simulink model "Hybridchargingstation"  (R2022a)
settings: Solver=ode23tb  StartTime=0.0  StopTime=20  RelTol=1e-3  EnableMultiTasking=on
undefined symbols (not defined in the file): Ion, Lithium
libraries: spsVoltageMeasurementLib x15, spsSeriesRLCBranchLib x9, spsIdealSwitchLib x9, spsDiodeLib x8, slpidlib x7, spsMeanLib x7, eePowerMeasurement x7, spsCurrentMeasurementLib x7, spsPWMGeneratorDCDCLib x4, spsMosfetLib x3, spsACVoltageSourceLib x3, spsBatteryLib x2
(part 1 of 2)
settings Model: Creator=kishor joshi  LastModifiedBy=Sri Charan Reddy
settings SolverCC: AlgebraicLoopSolver=TrustRegion
settings DataIOCC: ReturnWorkspaceOutputs=off
settings OptimizationCC: LifeSpan=inf
settings DebuggingCC: UnconnectedInputMsg=warning  UnconnectedOutputMsg=warning  UnconnectedLineMsg=warning  SFUnexpectedBacktrackingDiag=warning  SFNoUnconditionalDefaultTransitionDiag=warning  SFMachineParentedDataDiag=warning  ArithmeticOperatorsInVariantConditions=warning
settings SFSimCC: SimUseLocalCustomCode=off  CustomCodeUndefinedFunction=UseInterfaceOnly
settings RTWCC: RTWUseLocalCustomCode=off
settings CodeAppCC: StateflowObjectComments=on
settings GRTTargetCC: TargetLangStandard=C89/C90 (ANSI)
settings ConfigComp: CovMetricSettings=dw  CovSaveCumulativeToWorkspaceVar=on  CovSaveSingleToWorkspaceVar=on  CovExternalEMLEnable=off
settings SimscapeCC: SimscapeNormalizeSystem=off

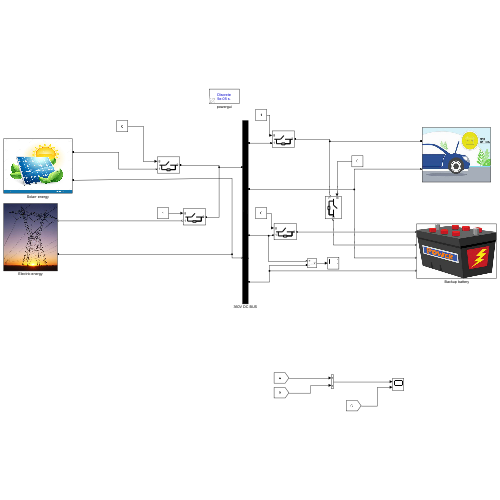
[thumbnail: Simulink's stored preview of the top-level diagram]
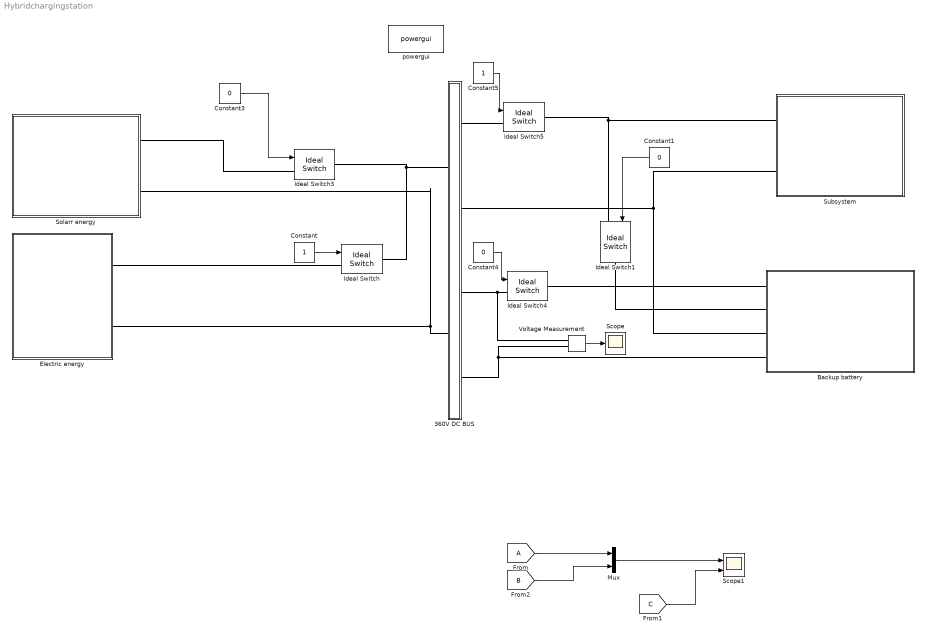
== system Hybridchargingstation ==
  " Backup battery" : Subsystem
      mask Display: image('C:\Users\Sri Charan Reddy\Downloads\OIP (1).jpg'); % Use "Edit Image" on toolstrip to change.
  360V DC BUS : Subsystem
  Constant : Constant
  Constant1 : Constant  Value=0
  Constant3 : Constant  Value=0
  Constant4 : Constant  Value=0
  Constant5 : Constant
  Electric energy : Subsystem
      mask Display: image('C:\Users\Sri Charan Reddy\Downloads\OIP.jpg'); % Use "Edit Image" on toolstrip to change.
  From : From  TagVisibility=global
  Ideal Switch{,1,3..5} (5 alike) : spsIdealSwitchLib/Ideal Switch  Ron=0.001  Lon=0  IC=0  Rs=1e5  Cs=inf  Measurements=off
  Mux : Mux  Inputs=2
      settings: DisplayOption=signals
  Scope : Scope
  Scope1 : Scope  NumInputPorts=2
  Solarr energy : Subsystem
      mask Display: image('C:\Users\Sri Charan Reddy\Downloads\solar-panel-green-energy-icon-vector-illustration-solar-panel-green-energy-icon-109072552.webp'); % Use "Edit Image" on toolstrip to change.
  Subsystem : Subsystem
      mask Display: image('C:\Users\Sri Charan Reddy\Downloads\OIP (2).jpg'); % Use "Edit Image" on toolstrip to change.
  Voltage Measurement : spsVoltageMeasurementLib/Voltage Measurement  PhasorSimulation=off  OutputType=Complex  PSBequivalent=0
  powergui : spspowerguiLib/powergui  Priority=1  SimulationMode=Discrete  SampleTime=50e-6  frequency=60  Iterations=50  frequencyindice=0  Pbase=100e6  ErrMax=1e-4  UnitsV=kV  UnitsW=MW  buscounter=0  FunctionMessages=off  echomessages=off  EnableUseOfTLC=off  CurrentSourceSwitches=off  DisableSnubberDevices=off  DisableRonSwitches=off  DisableVfSwitches=off  DisplayEquations=off  AutomaticDiscreteSolvers=off  SolverType=Tustin/Backward Euler (TBE)  Interpol=off  ExternalGateDelay=off  methode=off  Ts=100  x0status=blocks  SPID=on  SwTol=0  HookPort=off  NonlinearTolerance=1e-4  nMaxIteration=100  ContinueOnMaxIteration=off  RestoreLinks=warning  ResistiveCurrentMeasurement=off  Frange=[0:2:500]  Ylog=off  Xlog=on  ShowGrid=off  save=off  variable=ZData  structure=0  ZoomFFT=off  StartTime=0.0  cycles=1  DisplayStyle=1  fundamental=60  FreqAxis=off  MaxFrequency=1000  frequencyindicesteady=1  RmsSteady=1  display=off
  wires:
  Constant/1 -> Ideal Switch/1
  Constant3/1 -> Ideal Switch3/1
  Constant4/1 -> Ideal Switch4/1
  Constant5/1 -> Ideal Switch5/1
  Constant1/1 -> Ideal Switch1/1
  Voltage Measurement/1 -> Scope/1
  From/1 -> Mux/1
  [B] -> Mux/2
  Mux/1 -> Scope1/1
  [C] -> Scope1/2
  connections:
  360V DC BUS/LConn1 -- Ideal Switch3/RConn1 -- Ideal Switch/RConn1
  360V DC BUS/RConn2 -- Subsystem/LConn2 -- " Backup battery"/LConn3
  Ideal Switch4/LConn1 -- Voltage Measurement/LConn1 -- 360V DC BUS/RConn3
  360V DC BUS/RConn1 -- Ideal Switch5/LConn1
  Ideal Switch/LConn1 -- Electric energy/RConn1
  Solarr energy/RConn1 -- Ideal Switch3/LConn1
  Electric energy/RConn2 -- Solarr energy/RConn2 -- 360V DC BUS/LConn2
  Ideal Switch4/RConn1 -- " Backup battery"/LConn1
  Ideal Switch1/RConn1 -- " Backup battery"/LConn2
  360V DC BUS/RConn4 -- Voltage Measurement/LConn2 -- " Backup battery"/LConn4
  Ideal Switch1/LConn1 -- Subsystem/LConn1 -- Ideal Switch5/RConn1

== system Hybridchargingstation/ Backup battery ==
  Bidirectional buck-boost converter : Subsystem
      mask Display: image('C:\Users\Sri Charan Reddy\Downloads\Circuit-diagram-of-bidirectional-buck-boost-converter.png'); % Use "Edit Image" on toolstrip to change.
  + : PMIOPort  Side=Left
  2 : PMIOPort  Port=2  Side=Left
  S1 : PMIOPort  Port=3  Side=Left
  S : PMIOPort  Port=4  Side=Left
  connections:
  Bidirectional buck-boost converter/LConn2 -- S/RConn1
  Bidirectional buck-boost converter/LConn4 -- S1/RConn1
  Bidirectional buck-boost converter/LConn3 -- 2/RConn1
  Bidirectional buck-boost converter/LConn1 -- +/RConn1

== system Hybridchargingstation/360V DC BUS ==
  Connection Port : PMIOPort  Side=Left
  Vout- : PMIOPort  Port=2  Side=Left
  Conn5 : PMIOPort  Port=3  Side=Right
  Conn1 : PMIOPort  Port=4  Side=Right
  Conn2 : PMIOPort  Port=5  Side=Right
  Conn3 : PMIOPort  Port=6  Side=Right
  connections:
  Vout-/RConn1 -- Conn3/RConn1 -- Conn1/RConn1
  Connection Port/RConn1 -- Conn2/RConn1 -- Conn5/RConn1

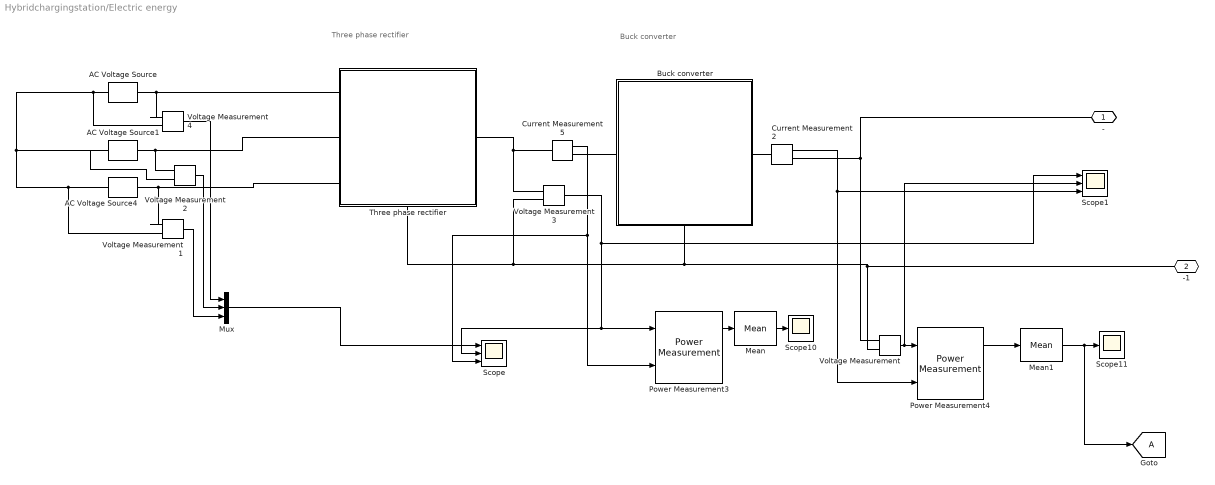
== system Hybridchargingstation/Electric energy ==
  note: Buck converter
  note: Three phase rectifier
  AC Voltage Source : spsACVoltageSourceLib/AC Voltage Source  Amplitude=325.5  Phase=0  Frequency=50  SampleTime=0  Measurements=None  BusType=swing  Pref=10e3  Qref=0  Qmin=-inf  Qmax=+inf
  AC Voltage Source1 : spsACVoltageSourceLib/AC Voltage Source  Amplitude=325.5  Phase=120  Frequency=50  SampleTime=0  Measurements=None  BusType=swing  Pref=10e3  Qref=0  Qmin=-inf  Qmax=+inf
  AC Voltage Source4 : spsACVoltageSourceLib/AC Voltage Source  Amplitude=325.5  Phase=240  Frequency=50  SampleTime=0  Measurements=None  BusType=swing  Pref=10e3  Qref=0  Qmin=-inf  Qmax=+inf
  Buck converter : Subsystem
      settings: PortSchema="{\"entries\":[{\"content\":{\"sides\":[{\"content\":{\"connectorIds\":[\"LConn1\"]},\"type\":\"ConnectorPlacement.EquallySpacedRectSide\",\"uuid\":\"d5439bf3-1a2a-4b74-ac5b-3787f53fe0e7\"},{\"content\":{\"connectorIds\":[\"RConn1\"],\"side\":\"RIGHT\"},\"type\":\"ConnectorPlacement.EquallySpacedRectSide\",\"uuid\":\"0cabc32d-cdfa-49eb-a496-5f16744d4e55\"},{\"content\":{\"connectorIds\":[],\"side\":\"TOP\"},\"type\":\"ConnectorPlacement.EquallySpacedRectSide\",\"uuid\":\"8a00a4d5-5aa0-4f1c-92a7-47fdc6fceede\"},{\"content\":{\"connectorIds\":[\"RConn2\"],\"side\":\"BOTTOM\"},\"type\":\"ConnectorPlacement.EquallySpacedRectSide\",\"uuid\":\"72676e0e-e154-49d7-9530-33720aeb54d2\"}]},\"type\":\"ConnectorPlacement.EquallySpacedConnector\",\"uuid\":\"34225297-7978-4460-82f7-cd42f07ac10d\"}],\"packageUris\":[\"http://schema.mathworks.com/mf0/Connector/R2020b\"],\"version\":\"1.0\"}"
      mask Display: image('C:\Users\Sri Charan Reddy\Downloads\OIP (3).jpg'); % Use "Edit Image" on toolstrip to change.
  Current Measurement2 : spsCurrentMeasurementLib/Current Measurement  PhasorSimulation=off  OutputType=Complex  PSBequivalent=0
  Current Measurement5 : spsCurrentMeasurementLib/Current Measurement  PhasorSimulation=off  OutputType=Complex  PSBequivalent=0
  Goto : Goto  TagVisibility=global
  Mean : spsMeanLib/Mean  Freq=50  Vinit=0  Ts=0
  Mean1 : spsMeanLib/Mean  Freq=50  Vinit=0  Ts=0
  Mux : Mux  Inputs=3
  Power Measurement3 : eePowerMeasurement/Power Measurement  LabelModeActiveChoice=Continuous  F=50  K=[0 ]  Ts=0
      settings: SourceProductBaseCode=PS
  Power Measurement4 : eePowerMeasurement/Power Measurement  LabelModeActiveChoice=Continuous  F=50  K=[0 ]  Ts=0
      settings: SourceProductBaseCode=PS
  Scope : Scope  NumInputPorts=3
  Scope1 : Scope  NumInputPorts=3
  Scope10 : Scope
  Scope11 : Scope
  Three phase rectifier : Subsystem
      settings: PortSchema="{\"entries\":[{\"content\":{\"sides\":[{\"content\":{\"connectorIds\":[\"LConn1\",\"LConn2\",\"LConn3\"]},\"type\":\"ConnectorPlacement.EquallySpacedRectSide\",\"uuid\":\"20f15a33-5136-48c0-8289-aa6a17724d94\"},{\"content\":{\"connectorIds\":[\"RConn1\"],\"side\":\"RIGHT\"},\"type\":\"ConnectorPlacement.EquallySpacedRectSide\",\"uuid\":\"ac3efbc5-b054-4a78-b49b-0a02bd728acf\"},{\"content\":{\"connectorIds\":[],\"side\":\"TOP\"},\"type\":\"ConnectorPlacement.EquallySpacedRectSide\",\"uuid\":\"8bb6768d-c71f-4225-afad-9830e861a3b7\"},{\"content\":{\"connectorIds\":[\"RConn2\"],\"side\":\"BOTTOM\"},\"type\":\"ConnectorPlacement.EquallySpacedRectSide\",\"uuid\":\"80e1a394-d96d-4650-a49c-4fe2462d5bbd\"}]},\"type\":\"ConnectorPlacement.EquallySpacedConnector\",\"uuid\":\"bddfc232-eb48-4920-a0a6-2caed26ef6d9\"}],\"packageUris\":[\"http://schema.mathworks.com/mf0/Connector/R2020b\"],\"version\":\"1.0\"}"
      mask Display: image('C:\Users\Sri Charan Reddy\Downloads\power97.gif'); % Use "Edit Image" on toolstrip to change.
  Voltage Measurement{,1..4} (5 alike) : spsVoltageMeasurementLib/Voltage Measurement  PhasorSimulation=off  OutputType=Complex  PSBequivalent=0
  - : PMIOPort  Side=Right
  -1 : PMIOPort  Port=2  Side=Right
  wires:
  Power Measurement4/1 -> Mean1/1
  Voltage Measurement/1 -> Scope1/2, Power Measurement4/1
  Current Measurement2/1 -> Scope1/3, Power Measurement4/2
  Current Measurement5/1 -> Scope/3, Power Measurement3/2
  Voltage Measurement3/1 -> Scope1/1, Scope/2, Power Measurement3/1
  Power Measurement3/1 -> Mean/1
  Mean/1 -> Scope10/1
  Mean1/1 -> Goto/1, Scope11/1
  Voltage Measurement4/1 -> Mux/1
  Voltage Measurement2/1 -> Mux/2
  Voltage Measurement1/1 -> Mux/3
  Mux/1 -> Scope/1
  connections:
  AC Voltage Source4/LConn1 -- Voltage Measurement1/LConn2 -- Voltage Measurement2/LConn2 -- AC Voltage Source1/LConn1 -- Voltage Measurement4/LConn2 -- AC Voltage Source/LConn1
  Voltage Measurement/LConn1 -- -/RConn1 -- Current Measurement2/RConn1
  Three phase rectifier/LConn3 -- Voltage Measurement1/LConn1 -- AC Voltage Source4/RConn1
  Three phase rectifier/RConn1 -- Current Measurement5/LConn1 -- Voltage Measurement3/LConn1
  AC Voltage Source1/RConn1 -- Voltage Measurement2/LConn1 -- Three phase rectifier/LConn2
  Voltage Measurement/LConn2 -- Buck converter/RConn2 -- Voltage Measurement3/LConn2 -- Three phase rectifier/RConn2 -- -1/RConn1
  AC Voltage Source/RConn1 -- Voltage Measurement4/LConn1 -- Three phase rectifier/LConn1
  Current Measurement2/LConn1 -- Buck converter/LConn1
  Buck converter/RConn1 -- Current Measurement5/RConn1

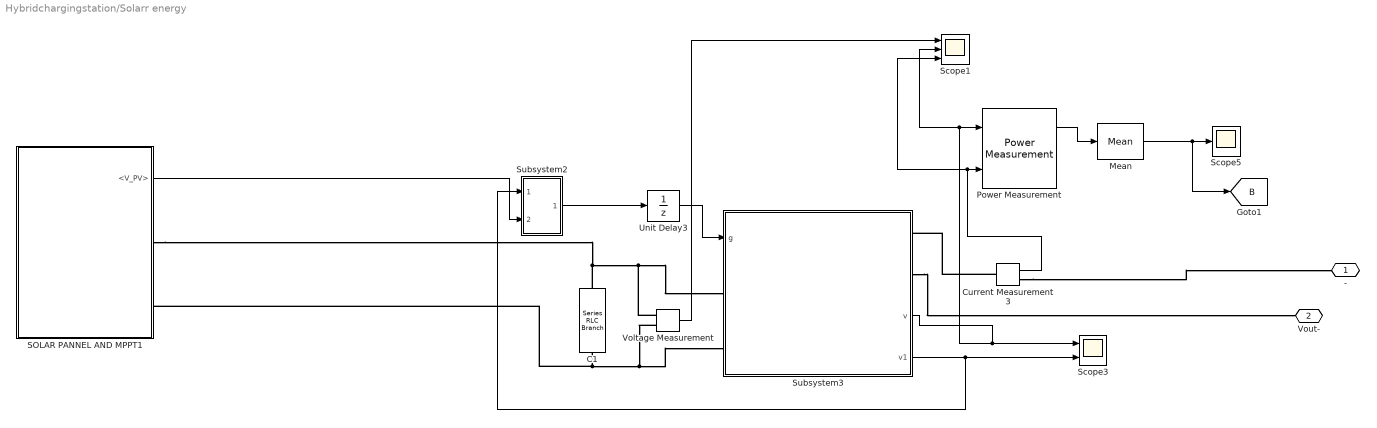
== system Hybridchargingstation/Solarr energy ==
  C1 : spsSeriesRLCBranchLib/Series RLC Branch  LConnTagsString=__new0  RConnTagsString=__new0  BranchType=C  Resistance=1  Inductance=1e-3  SetiL0=off  InitialCurrent=0  Capacitance=2300e-6  Setx0=off  InitialVoltage=0  Measurements=None
  Current Measurement3 : spsCurrentMeasurementLib/Current Measurement  PhasorSimulation=off  OutputType=Complex  PSBequivalent=0
  Mean : spsMeanLib/Mean  Freq=50  Vinit=0  Ts=0
  Power Measurement : eePowerMeasurement/Power Measurement  LabelModeActiveChoice=Continuous  F=50  K=[0 ]  Ts=0
      settings: SourceProductBaseCode=PS
  SOLAR PANNEL AND MPPT1 : Subsystem
      mask Display: image('C:\Users\Sri Charan Reddy\Downloads\solar-power-panel-concept-animation_m1n8aunv_thumbnail-1080_01.png'); % Use "Edit Image" on toolstrip to change.
  Scope1 : Scope  NumInputPorts=3
  Scope3 : Scope  NumInputPorts=2
  Scope5 : Scope
  Subsystem2 : Subsystem
  Subsystem3 : Subsystem
      settings: PortSchema="{\"entries\":[{\"content\":{\"sides\":[{\"content\":{\"connectorIds\":[\"In1\",\"LConn1\",\"LConn2\"]},\"type\":\"ConnectorPlacement.EquallySpacedRectSide\",\"uuid\":\"b486ab45-7f3f-4730-9797-5751a0205d1a\"},{\"content\":{\"connectorIds\":[\"RConn1\",\"RConn2\",\"Out1\",\"Out2\"],\"side\":\"RIGHT\"},\"type\":\"ConnectorPlacement.EquallySpacedRectSide\",\"uuid\":\"d803486f-6150-4425-aefb-53dd6f789c0c\"},{\"content\":{\"connectorIds\":[],\"side\":\"TOP\"},\"type\":\"ConnectorPlacement.EquallySpacedRectSide\",\"uuid\":\"185bad64-41d0-46fa-a4c0-3fb5674fae4a\"},{\"content\":{\"connectorIds\":[],\"side\":\"BOTTOM\"},\"type\":\"ConnectorPlacement.EquallySpacedRectSide\",\"uuid\":\"7050c488-9833-477f-87d1-db99736a9e7e\"}]},\"type\":\"ConnectorPlacement.EquallySpacedConnector\",\"uuid\":\"2c79cd5d-622c-43de-b277-67401261fd36\"}],\"packageUris\":[\"http://schema.mathworks.com/mf0/Connector/R2020b\"],\"version\":\"1.0\"}"
      mask Display: image('C:\Users\Sri Charan Reddy\Downloads\OIP (4).jpg'); % Use "Edit Image" on toolstrip to change.
  Unit Delay3 : UnitDelay  SampleTime=-1
  Voltage Measurement : spsVoltageMeasurementLib/Voltage Measurement  PhasorSimulation=off  OutputType=Complex  PSBequivalent=0
  - : PMIOPort  Side=Right
  Vout- : PMIOPort  Port=2  Side=Right
  tag scope: B=global
  wires:
  Subsystem3/1(v) -> Scope3/1, Scope1/2, Power Measurement/1
  Unit Delay3/1 -> Subsystem3/1(g)
  SOLAR PANNEL AND MPPT1/1(<V_PV>) -> Subsystem2/2(Vdc1)
  Subsystem2/1(Out2) -> Unit Delay3/1
  Subsystem3/2(v1) -> Subsystem2/1(Vdc), Scope3/2
  Power Measurement/1 -> Mean/1
  Current Measurement3/1 -> Scope1/3, Power Measurement/2
  Mean/1 -> [B], Scope5/1
  Voltage Measurement/1 -> Scope1/1
  connections:
  C1/RConn1 -- SOLAR PANNEL AND MPPT1/RConn1 -- Voltage Measurement/LConn1 -- Subsystem3/LConn1
  Subsystem3/RConn2 -- Vout-/RConn1
  Current Measurement3/LConn1 -- Subsystem3/RConn1
  SOLAR PANNEL AND MPPT1/RConn2 -- C1/LConn1 -- Voltage Measurement/LConn2 -- Subsystem3/LConn2
  Current Measurement3/RConn1 -- -/RConn1

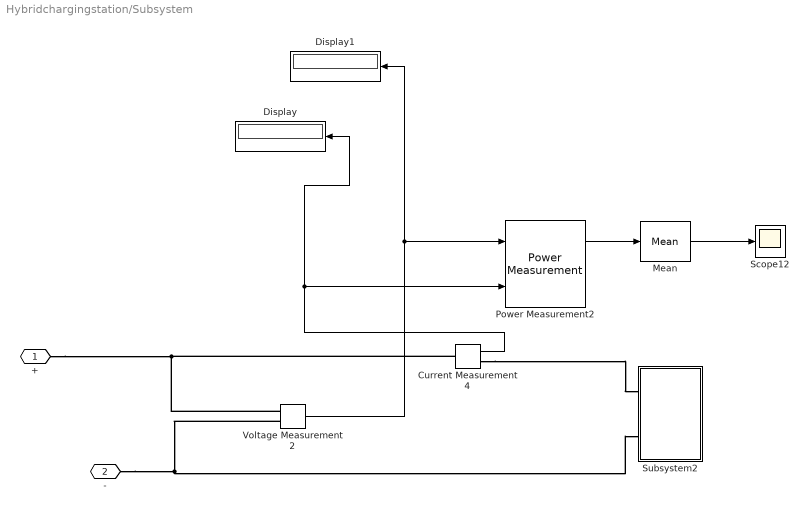
== system Hybridchargingstation/Subsystem ==
  Current Measurement4 : spsCurrentMeasurementLib/Current Measurement  PhasorSimulation=off  OutputType=Complex  PSBequivalent=0
  Display : Display
  Display1 : Display
  Mean : spsMeanLib/Mean  Freq=60  Vinit=0  Ts=0
  Power Measurement2 : eePowerMeasurement/Power Measurement  LabelModeActiveChoice=Continuous  F=50  K=[0]  Ts=0
      settings: SourceProductBaseCode=PS
  Scope12 : Scope
  Subsystem2 : Subsystem
  Voltage Measurement2 : spsVoltageMeasurementLib/Voltage Measurement  PhasorSimulation=off  OutputType=Complex  PSBequivalent=0
  + : PMIOPort  Side=Left
  - : PMIOPort  Port=2  Side=Left
  wires:
  Voltage Measurement2/1 -> Display1/1, Power Measurement2/1
  Current Measurement4/1 -> Display/1, Power Measurement2/2
  Power Measurement2/1 -> Mean/1
  Mean/1 -> Scope12/1
  connections:
  Current Measurement4/LConn1 -- Voltage Measurement2/LConn1 -- +/RConn1
  Voltage Measurement2/LConn2 -- -/RConn1 -- Subsystem2/LConn2
  Current Measurement4/RConn1 -- Subsystem2/LConn1

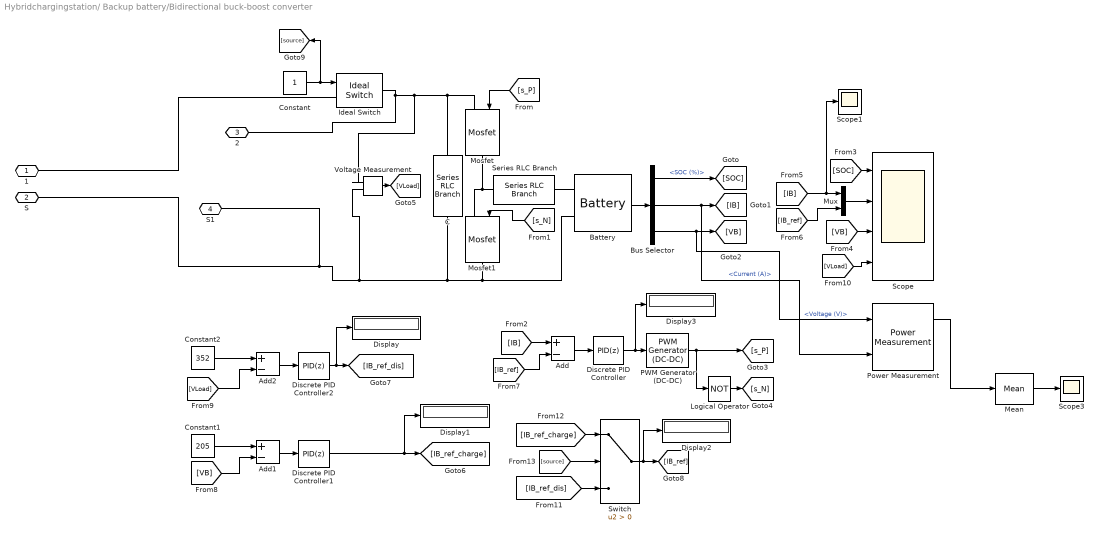
== system Hybridchargingstation/ Backup battery/Bidirectional buck-boost converter ==
  Add : Sum  Inputs=+-
  Add1 : Sum  Inputs=+-
  Add2 : Sum  Inputs=+-
  Battery : spsBatteryLib/Battery  BatType=Lithium-Ion  ShowTempParam=off  ThermalPreset=no  ShowAgeParam=off  NomV=200  NomQ=50  SOC=45  Batt_Tr=1  PresetModel=on  MaxQ=50  MinV=150  FullV=232.7974  Dis_rate=21.7391  R=0.04  Normal_OP=45.2174  expZone="[216.0772      2.456522]"  current=[6.5 13 32.5]  Units=Time  Tci=20  NomT=20  T2=-30  MaxQ2=4.8  FullV2=7.1  Normal_OP2=5.655  expZone2="[6.58           1]"  Rca=0.6  ti=2000  Dp=0  Neq0=0  Tsim=1e6  Ta1=25  Qeol=5.4*0.9  Reol=0.013333*1.2  Char_age=[2.3478, 3]  Dis_age=[2.3478, 10]  N1=1500  N2=10500  N3=1000  N4=1400  Ta2=45  N5=950
  Bus Selector : BusSelector  OutputSignals=SOC (%),Current (A),Voltage (V)
  C : spsSeriesRLCBranchLib/Series RLC Branch  LConnTagsString=__new0  RConnTagsString=__new0  BranchType=RC  Resistance=0.001  Inductance=5.76e-4  SetiL0=off  InitialCurrent=0  Capacitance=1000e-6  Setx0=off  InitialVoltage=0  Measurements=None
  Constant : Constant
  Constant1 : Constant  Value=205
  Constant2 : Constant  Value=352
  Discrete PID Controller : slpidlib/PID Controller  Controller=PID  Form=Parallel  TimeDomain=Discrete-time  UseExternalTs=off  SampleTime=-1  IntegratorMethod=Forward Euler  FilterMethod=Forward Euler  ControllerParametersSource=internal  P=0.05  I=0.01  UseKiTs=off  D=0  N=100  UseFilter=on  TunerSelectOption=Transfer Function Based (PID Tuner App)  InitialConditionSource=internal  InitialConditionForIntegrator=0  InitialConditionForFilter=0  DifferentiatorICPrevScaledInput=0  ExternalReset=none  TrackingMode=off  Kt=1  LimitOutput=off  SatLimitsSource=internal  UpperSaturationLimit=inf  LowerSaturationLimit=-inf  LinearizeAsGain=off  AntiWindupMode=none  Kb=1  POutMin=[]  POutMax=[]  IOutMin=[]  IOutMax=[]  DOutMin=[]  DOutMax=[]  NOutMin=[]  NOutMax=[]  SumOutMin=[]  SumOutMax=[]  SaturationOutMin=[]  SaturationOutMax=[]  PParamMin=[]  PParamMax=[]  IParamMin=[]  IParamMax=[]  DParamMin=[]  DParamMax=[]  NParamMin=[]  NParamMax=[]  KbParamMin=[]  KbParamMax=[]  KtParamMin=[]  KtParamMax=[]  KbOutMin=[]  KbOutMax=[]  KtOutMin=[]  KtOutMax=[]  IntegratorOutMin=[]  IntegratorOutMax=[]  FilterOutMin=[]  FilterOutMax=[]  SumI1OutMin=[]  SumI1OutMax=[]  SumI2OutMin=[]  SumI2OutMax=[]  SumI3OutMin=[]  SumI3OutMax=[]  SumI4OutMin=[]  SumI4OutMax=[]  SumDOutMin=[]  SumDOutMax=[]  DifferentiatorOutMin=[]  DifferentiatorOutMax=[]  FilterDiffOutCoefMin=[]  FilterDiffOutCoefMax=[]  ReciprocalOutMin=[]  ReciprocalOutMax=[]  SumDenOutMin=[]  SumDenOutMax=[]  SumNumOutMin=[]  SumNumOutMax=[]  DivideOutMin=[]  DivideOutMax=[]  UdiffTsProdOutMin=[]  UdiffTsProdOutMax=[]  NTsProdOutMin=[]  NTsProdOutMax=[]  UintegralTsProdOutMin=[]  UintegralTsProdOutMax=[]  UngainTsProdOutMin=[]  UngainTsProdOutMax=[]  IntegratorContinuousStateAttributes=''  IntegratorStateMustResolveToSignalObject=off  IntegratorRTWStateStorageClass=Auto  FilterContinuousStateAttributes=''  FilterStateMustResolveToSignalObject=off  FilterRTWStateStorageClass=Auto  ParallelPVariant=InternalParameters  IdealPVariant=Disabled  IVariant=InternalParameters  DVariant=InternalParameters  IntegratorVariant=Discrete  SatVariant=Disabled  AWVariant=Passthrough  PCopyVariant=Disabled  TRVariant=Disabled  FdbkBlocksVariant=Forward  IdealPFdbkVariant=Disabled  SatFdbkVariant=Disabled  DerivativeFilterVariant=ForwardEulerFilter  NVariant=InternalParameters  NCopyVariant=Disabled  FilterICVariant=InternalICsFilter  IntegratorICVariant=InternalICs  ExternalResetVariant=Disabled  TRSumVariant=Passthrough  SumFdbkVariant=Disabled  SumVariant=Sum_PID  TsampFilterVariant=InternalTs  TsampNgainVariant=Passthrough  TsampIntegralVariant=Passthrough  ExternalSaturationOutDataTypeStr=Inherit: Same as second input  aMode=0
  Discrete PID Controller1 : slpidlib/PID Controller  Controller=PID  Form=Parallel  TimeDomain=Discrete-time  UseExternalTs=off  SampleTime=-1  IntegratorMethod=Forward Euler  FilterMethod=Forward Euler  ControllerParametersSource=internal  P=2.8  I=0.001  UseKiTs=off  D=0  N=100  UseFilter=on  TunerSelectOption=Transfer Function Based (PID Tuner App)  InitialConditionSource=internal  InitialConditionForIntegrator=0  InitialConditionForFilter=0  DifferentiatorICPrevScaledInput=0  ExternalReset=none  TrackingMode=off  Kt=1  LimitOutput=off  SatLimitsSource=internal  UpperSaturationLimit=inf  LowerSaturationLimit=-inf  LinearizeAsGain=off  AntiWindupMode=none  Kb=1  POutMin=[]  POutMax=[]  IOutMin=[]  IOutMax=[]  DOutMin=[]  DOutMax=[]  NOutMin=[]  NOutMax=[]  SumOutMin=[]  SumOutMax=[]  SaturationOutMin=[]  SaturationOutMax=[]  PParamMin=[]  PParamMax=[]  IParamMin=[]  IParamMax=[]  DParamMin=[]  DParamMax=[]  NParamMin=[]  NParamMax=[]  KbParamMin=[]  KbParamMax=[]  KtParamMin=[]  KtParamMax=[]  KbOutMin=[]  KbOutMax=[]  KtOutMin=[]  KtOutMax=[]  IntegratorOutMin=[]  IntegratorOutMax=[]  FilterOutMin=[]  FilterOutMax=[]  SumI1OutMin=[]  SumI1OutMax=[]  SumI2OutMin=[]  SumI2OutMax=[]  SumI3OutMin=[]  SumI3OutMax=[]  SumI4OutMin=[]  SumI4OutMax=[]  SumDOutMin=[]  SumDOutMax=[]  DifferentiatorOutMin=[]  DifferentiatorOutMax=[]  FilterDiffOutCoefMin=[]  FilterDiffOutCoefMax=[]  ReciprocalOutMin=[]  ReciprocalOutMax=[]  SumDenOutMin=[]  SumDenOutMax=[]  SumNumOutMin=[]  SumNumOutMax=[]  DivideOutMin=[]  DivideOutMax=[]  UdiffTsProdOutMin=[]  UdiffTsProdOutMax=[]  NTsProdOutMin=[]  NTsProdOutMax=[]  UintegralTsProdOutMin=[]  UintegralTsProdOutMax=[]  UngainTsProdOutMin=[]  UngainTsProdOutMax=[]  IntegratorContinuousStateAttributes=''  IntegratorStateMustResolveToSignalObject=off  IntegratorRTWStateStorageClass=Auto  FilterContinuousStateAttributes=''  FilterStateMustResolveToSignalObject=off  FilterRTWStateStorageClass=Auto  ParallelPVariant=InternalParameters  IdealPVariant=Disabled  IVariant=InternalParameters  DVariant=InternalParameters  IntegratorVariant=Discrete  SatVariant=Disabled  AWVariant=Passthrough  PCopyVariant=Disabled  TRVariant=Disabled  FdbkBlocksVariant=Forward  IdealPFdbkVariant=Disabled  SatFdbkVariant=Disabled  DerivativeFilterVariant=ForwardEulerFilter  NVariant=InternalParameters  NCopyVariant=Disabled  FilterICVariant=InternalICsFilter  IntegratorICVariant=InternalICs  ExternalResetVariant=Disabled  TRSumVariant=Passthrough  SumFdbkVariant=Disabled  SumVariant=Sum_PID  TsampFilterVariant=InternalTs  TsampNgainVariant=Passthrough  TsampIntegralVariant=Passthrough  ExternalSaturationOutDataTypeStr=Inherit: Same as second input  aMode=0
  Discrete PID Controller2 : slpidlib/PID Controller  Controller=PID  Form=Parallel  TimeDomain=Discrete-time  UseExternalTs=off  SampleTime=-1  IntegratorMethod=Forward Euler  FilterMethod=Forward Euler  ControllerParametersSource=internal  P=1  I=0.5  UseKiTs=off  D=0  N=100  UseFilter=on  TunerSelectOption=Transfer Function Based (PID Tuner App)  InitialConditionSource=internal  InitialConditionForIntegrator=0  InitialConditionForFilter=0  DifferentiatorICPrevScaledInput=0  ExternalReset=none  TrackingMode=off  Kt=1  LimitOutput=off  SatLimitsSource=internal  UpperSaturationLimit=inf  LowerSaturationLimit=-inf  LinearizeAsGain=off  AntiWindupMode=none  Kb=1  POutMin=[]  POutMax=[]  IOutMin=[]  IOutMax=[]  DOutMin=[]  DOutMax=[]  NOutMin=[]  NOutMax=[]  SumOutMin=[]  SumOutMax=[]  SaturationOutMin=[]  SaturationOutMax=[]  PParamMin=[]  PParamMax=[]  IParamMin=[]  IParamMax=[]  DParamMin=[]  DParamMax=[]  NParamMin=[]  NParamMax=[]  KbParamMin=[]  KbParamMax=[]  KtParamMin=[]  KtParamMax=[]  KbOutMin=[]  KbOutMax=[]  KtOutMin=[]  KtOutMax=[]  IntegratorOutMin=[]  IntegratorOutMax=[]  FilterOutMin=[]  FilterOutMax=[]  SumI1OutMin=[]  SumI1OutMax=[]  SumI2OutMin=[]  SumI2OutMax=[]  SumI3OutMin=[]  SumI3OutMax=[]  SumI4OutMin=[]  SumI4OutMax=[]  SumDOutMin=[]  SumDOutMax=[]  DifferentiatorOutMin=[]  DifferentiatorOutMax=[]  FilterDiffOutCoefMin=[]  FilterDiffOutCoefMax=[]  ReciprocalOutMin=[]  ReciprocalOutMax=[]  SumDenOutMin=[]  SumDenOutMax=[]  SumNumOutMin=[]  SumNumOutMax=[]  DivideOutMin=[]  DivideOutMax=[]  UdiffTsProdOutMin=[]  UdiffTsProdOutMax=[]  NTsProdOutMin=[]  NTsProdOutMax=[]  UintegralTsProdOutMin=[]  UintegralTsProdOutMax=[]  UngainTsProdOutMin=[]  UngainTsProdOutMax=[]  IntegratorContinuousStateAttributes=''  IntegratorStateMustResolveToSignalObject=off  IntegratorRTWStateStorageClass=Auto  FilterContinuousStateAttributes=''  FilterStateMustResolveToSignalObject=off  FilterRTWStateStorageClass=Auto  ParallelPVariant=InternalParameters  IdealPVariant=Disabled  IVariant=InternalParameters  DVariant=InternalParameters  IntegratorVariant=Discrete  SatVariant=Disabled  AWVariant=Passthrough  PCopyVariant=Disabled  TRVariant=Disabled  FdbkBlocksVariant=Forward  IdealPFdbkVariant=Disabled  SatFdbkVariant=Disabled  DerivativeFilterVariant=ForwardEulerFilter  NVariant=InternalParameters  NCopyVariant=Disabled  FilterICVariant=InternalICsFilter  IntegratorICVariant=InternalICs  ExternalResetVariant=Disabled  TRSumVariant=Passthrough  SumFdbkVariant=Disabled  SumVariant=Sum_PID  TsampFilterVariant=InternalTs  TsampNgainVariant=Passthrough  TsampIntegralVariant=Passthrough  ExternalSaturationOutDataTypeStr=Inherit: Same as second input  aMode=0
  Display{,1..3} (4 alike) : Display
  Ideal Switch : spsIdealSwitchLib/Ideal Switch  Ron=0.001  Lon=0  IC=0  Rs=1e5  Cs=inf  Measurements=off
  Logical Operator : Logic  Operator=NOT  AllPortsSameDT=off  OutDataTypeStr=boolean
  Mean : spsMeanLib/Mean  Freq=50  Vinit=0  Ts=0
  Mosfet : spsMosfetLib/Mosfet  Ron=0.1  Lon=0  Rd=0.01  Vfd=0  IC=0  Rs=1e5  Cs=inf  Measurements=off
  Mosfet1 : spsMosfetLib/Mosfet  Ron=0.1  Lon=0  Rd=0.01  Vfd=0  IC=0  Rs=1e5  Cs=inf  Measurements=off
  Mux : Mux  Inputs=2
  PWM Generator (DC-DC) : spsPWMGeneratorDCDCLib/PWM Generator (DC-DC)  Fsw=10e3  Ts=5e-6
  Power Measurement : eePowerMeasurement/Power Measurement  LabelModeActiveChoice=Continuous  F=50  K=[0 ]  Ts=0
      settings: SourceProductBaseCode=PS
  Scope : Scope  NumInputPorts=4
  Scope1 : Scope
  Scope3 : Scope
  Series RLC Branch : spsSeriesRLCBranchLib/Series RLC Branch  LConnTagsString=__new0  RConnTagsString=__new0  BranchType=RL  Resistance=0.05  Inductance=576e-4  SetiL0=off  InitialCurrent=0  Capacitance=1e-6  Setx0=off  InitialVoltage=0  Measurements=None
  Switch : Switch  Criteria=u2 > Threshold  SaturateOnIntegerOverflow=off  InputSameDT=off
  Voltage Measurement : spsVoltageMeasurementLib/Voltage Measurement  PhasorSimulation=off  OutputType=Complex  PSBequivalent=0
  1 : PMIOPort  Side=Left
  S : PMIOPort  Port=2  Side=Left
  2 : PMIOPort  Port=3  Side=Left
  S1 : PMIOPort  Port=4  Side=Left
  wires:
  Discrete PID Controller1/1 -> Display1/1, [IB_ref_charge]
  Add/1 -> Discrete PID Controller/1
  [s_N] -> Mosfet1/1
  Discrete PID Controller2/1 -> Display/1, [IB_ref_dis]
  Constant/1 -> [source], Ideal Switch/1
  Logical Operator/1 -> [s_N]
  [IB] -> Scope1/1, Mux/1
  [s_P] -> Mosfet/1
  Discrete PID Controller/1 -> Display3/1, PWM Generator (DC-DC)/1
  Add1/1 -> Discrete PID Controller1/1
  Bus Selector/1 -> [SOC]  "<SOC (%)>"
  [source] -> Switch/2
  Battery/1 -> Bus Selector/1
  Add2/1 -> Discrete PID Controller2/1
  Constant1/1 -> Add1/1
  [IB_ref_dis] -> Switch/3
  Bus Selector/2 -> Power Measurement/2, [IB]  "<Current (A)>"
  [IB] -> Add/1
  [SOC] -> Scope/1
  [VB] -> Scope/3
  PWM Generator (DC-DC)/1 -> [s_P], Logical Operator/1
  Bus Selector/3 -> Power Measurement/1, [VB]  "<Voltage (V)>"
  Constant2/1 -> Add2/1
  [VB] -> Add1/2
  [IB_ref] -> Mux/2
  [VLoad] -> Scope/4
  Voltage Measurement/1 -> [VLoad]
  Switch/1 -> Display2/1, [IB_ref]
  [VLoad] -> Add2/2
  Mux/1 -> Scope/2
  [IB_ref_charge] -> Switch/1
  [IB_ref] -> Add/2
  Power Measurement/1 -> Mean/1
  Mean/1 -> Scope3/1
  connections:
  Voltage Measurement/LConn2 -- S1/RConn1 -- S/RConn1 -- C/RConn1 -- Battery/LConn2 -- Mosfet1/RConn1
  Mosfet/RConn1 -- Series RLC Branch/LConn1 -- Mosfet1/LConn1
  C/LConn1 -- Voltage Measurement/LConn1 -- 2/RConn1 -- Ideal Switch/RConn1 -- Mosfet/LConn1
  Series RLC Branch/RConn1 -- Battery/LConn1
  1/RConn1 -- Ideal Switch/LConn1

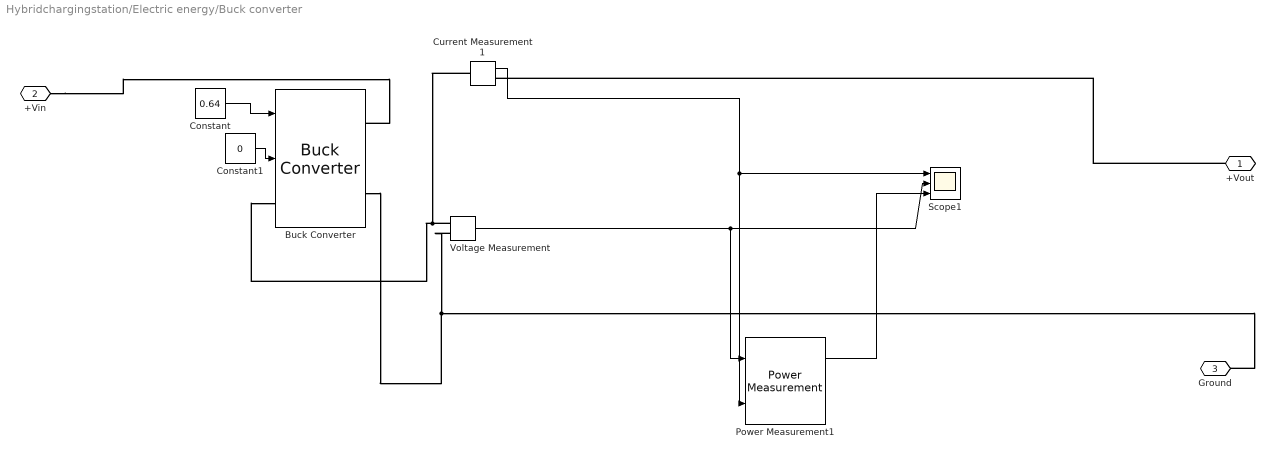
== system Hybridchargingstation/Electric energy/Buck converter ==
  Buck Converter : spsBuckConverterLib/Buck Converter  ModelType=Average model (D-controlled)  Ron=1e-3  Rs=1e6  Cs=inf  Vforward=[0,0]  Ron_Diode=1e-3  Rs_Diode=1e6  Cs_Diode=inf  Vf_Diode=1e-3  Rs_CurrentSource=inf  Ron_ACsource=1e-3
      settings: SourceProductBaseCode=PS
  Constant : Constant  Value=0.64
  Constant1 : Constant  Value=0
  Current Measurement1 : spsCurrentMeasurementLib/Current Measurement  PhasorSimulation=off  OutputType=Complex  PSBequivalent=0
  Power Measurement1 : eePowerMeasurement/Power Measurement  LabelModeActiveChoice=Continuous  F=50  K=[0 1 2 3]  Ts=0
      settings: SourceProductBaseCode=PS
  Scope1 : Scope  NumInputPorts=3
  Voltage Measurement : spsVoltageMeasurementLib/Voltage Measurement  PhasorSimulation=off  OutputType=Complex  PSBequivalent=0
  +Vout : PMIOPort  Side=Left
  +Vin : PMIOPort  Port=2  Side=Right
  Ground : PMIOPort  Port=3  Side=Right
  wires:
  Voltage Measurement/1 -> Power Measurement1/1, Scope1/2
  Current Measurement1/1 -> Power Measurement1/2, Scope1/1
  Constant1/1 -> Buck Converter/2
  Power Measurement1/1 -> Scope1/3
  Constant/1 -> Buck Converter/1
  connections:
  Voltage Measurement/LConn1 -- Current Measurement1/LConn1 -- Buck Converter/LConn1
  Voltage Measurement/LConn2 -- Buck Converter/RConn2 -- Ground/RConn1
  +Vout/RConn1 -- Current Measurement1/RConn1
  +Vin/RConn1 -- Buck Converter/RConn1

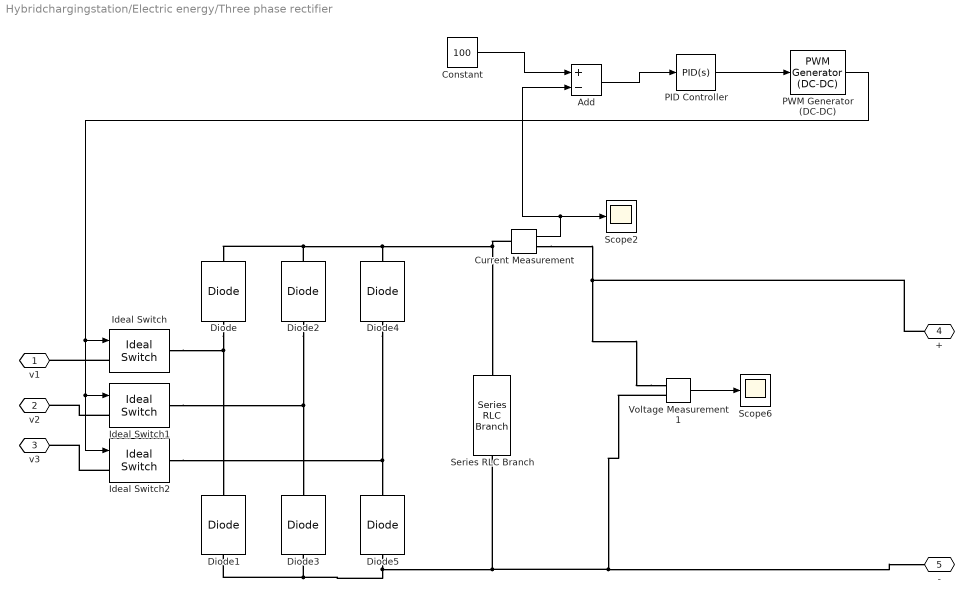
== system Hybridchargingstation/Electric energy/Three phase rectifier ==
  Add : Sum  Inputs=+-
  Constant : Constant  Value=100
  Current Measurement : spsCurrentMeasurementLib/Current Measurement  PhasorSimulation=off  OutputType=Complex  PSBequivalent=0
  Diode{,1..5} (6 alike) : spsDiodeLib/Diode  Ron=0.001  Lon=0  Vf=0.8  IC=0  UseSnubber=0  Rs=500  Cs=250e-9  Measurements=off
  Ideal Switch : spsIdealSwitchLib/Ideal Switch  Ron=0.001  Lon=0  IC=0  Rs=1e5  Cs=inf  Measurements=off
  Ideal Switch1 : spsIdealSwitchLib/Ideal Switch  Ron=0.001  Lon=0  IC=0  Rs=1e5  Cs=inf  Measurements=off
  Ideal Switch2 : spsIdealSwitchLib/Ideal Switch  Ron=0.001  Lon=0  IC=0  Rs=1e5  Cs=inf  Measurements=off
  PID Controller : slpidlib/PID Controller  Controller=PID  Form=Parallel  TimeDomain=Continuous-time  UseExternalTs=off  SampleTime=-1  IntegratorMethod=Forward Euler  FilterMethod=Forward Euler  ControllerParametersSource=internal  P=0.01  I=100  UseKiTs=off  D=0  N=100  UseFilter=on  TunerSelectOption=Transfer Function Based (PID Tuner App)  InitialConditionSource=internal  InitialConditionForIntegrator=0  InitialConditionForFilter=0  DifferentiatorICPrevScaledInput=0  ExternalReset=none  TrackingMode=off  Kt=1  LimitOutput=off  SatLimitsSource=internal  UpperSaturationLimit=inf  LowerSaturationLimit=-inf  LinearizeAsGain=on  AntiWindupMode=none  Kb=1  POutMin=[]  POutMax=[]  IOutMin=[]  IOutMax=[]  DOutMin=[]  DOutMax=[]  NOutMin=[]  NOutMax=[]  SumOutMin=[]  SumOutMax=[]  SaturationOutMin=[]  SaturationOutMax=[]  PParamMin=[]  PParamMax=[]  IParamMin=[]  IParamMax=[]  DParamMin=[]  DParamMax=[]  NParamMin=[]  NParamMax=[]  KbParamMin=[]  KbParamMax=[]  KtParamMin=[]  KtParamMax=[]  KbOutMin=[]  KbOutMax=[]  KtOutMin=[]  KtOutMax=[]  IntegratorOutMin=[]  IntegratorOutMax=[]  FilterOutMin=[]  FilterOutMax=[]  SumI1OutMin=[]  SumI1OutMax=[]  SumI2OutMin=[]  SumI2OutMax=[]  SumI3OutMin=[]  SumI3OutMax=[]  SumI4OutMin=[]  SumI4OutMax=[]  SumDOutMin=[]  SumDOutMax=[]  DifferentiatorOutMin=[]  DifferentiatorOutMax=[]  FilterDiffOutCoefMin=[]  FilterDiffOutCoefMax=[]  ReciprocalOutMin=[]  ReciprocalOutMax=[]  SumDenOutMin=[]  SumDenOutMax=[]  SumNumOutMin=[]  SumNumOutMax=[]  DivideOutMin=[]  DivideOutMax=[]  UdiffTsProdOutMin=[]  UdiffTsProdOutMax=[]  NTsProdOutMin=[]  NTsProdOutMax=[]  UintegralTsProdOutMin=[]  UintegralTsProdOutMax=[]  UngainTsProdOutMin=[]  UngainTsProdOutMax=[]  IntegratorContinuousStateAttributes=''  IntegratorStateMustResolveToSignalObject=off  IntegratorRTWStateStorageClass=Auto  FilterContinuousStateAttributes=''  FilterStateMustResolveToSignalObject=off  FilterRTWStateStorageClass=Auto  ParallelPVariant=InternalParameters  IdealPVariant=Disabled  IVariant=InternalParameters  DVariant=InternalParameters  IntegratorVariant=Continuous  SatVariant=Disabled  AWVariant=Passthrough  PCopyVariant=Disabled  TRVariant=Disabled  FdbkBlocksVariant=Forward  IdealPFdbkVariant=Disabled  SatFdbkVariant=Disabled  DerivativeFilterVariant=ContFilter  NVariant=InternalParameters  NCopyVariant=Disabled  FilterICVariant=InternalICsFilter  IntegratorICVariant=InternalICs  ExternalResetVariant=Disabled  TRSumVariant=Passthrough  SumFdbkVariant=Disabled  SumVariant=Sum_PID  TsampFilterVariant=InternalTs  TsampNgainVariant=Passthrough  TsampIntegralVariant=Passthrough  ExternalSaturationOutDataTypeStr=Inherit: Same as second input  aMode=0
  PWM Generator (DC-DC) : spsPWMGeneratorDCDCLib/PWM Generator (DC-DC)  Fsw=100000  Ts=0
  Scope2 : Scope
  Scope6 : Scope
  Series RLC Branch : spsSeriesRLCBranchLib/Series RLC Branch  LConnTagsString=__new0  RConnTagsString=__new0  BranchType=C  Resistance=1  Inductance=1e-3  SetiL0=off  InitialCurrent=0  Capacitance=1000e-3  Setx0=off  InitialVoltage=0  Measurements=Branch voltage
  Voltage Measurement1 : spsVoltageMeasurementLib/Voltage Measurement  PhasorSimulation=off  OutputType=Complex  PSBequivalent=0
  v1 : PMIOPort  Side=Left
  v2 : PMIOPort  Port=2  Side=Left
  v3 : PMIOPort  Port=3  Side=Left
  + : PMIOPort  Port=4  Side=Right
  - : PMIOPort  Port=5  Side=Right
  wires:
  Voltage Measurement1/1 -> Scope6/1
  Current Measurement/1 -> Add/2, Scope2/1
  Constant/1 -> Add/1
  Add/1 -> PID Controller/1
  PID Controller/1 -> PWM Generator (DC-DC)/1
  PWM Generator (DC-DC)/1 -> Ideal Switch1/1, Ideal Switch2/1, Ideal Switch/1
  connections:
  Diode5/LConn1 -- -/RConn1 -- Voltage Measurement1/LConn2 -- Series RLC Branch/RConn1 -- Diode1/LConn1 -- Diode3/LConn1
  Diode2/LConn1 -- Diode3/RConn1 -- Ideal Switch1/RConn1
  Diode4/LConn1 -- Diode5/RConn1 -- Ideal Switch2/RConn1
  Diode2/RConn1 -- Current Measurement/LConn1 -- Series RLC Branch/LConn1 -- Diode4/RConn1 -- Diode/RConn1
  Voltage Measurement1/LConn1 -- +/RConn1 -- Current Measurement/RConn1
  Diode/LConn1 -- Diode1/RConn1 -- Ideal Switch/RConn1
  Ideal Switch/LConn1 -- v1/RConn1
  Ideal Switch1/LConn1 -- v2/RConn1
  Ideal Switch2/LConn1 -- v3/RConn1

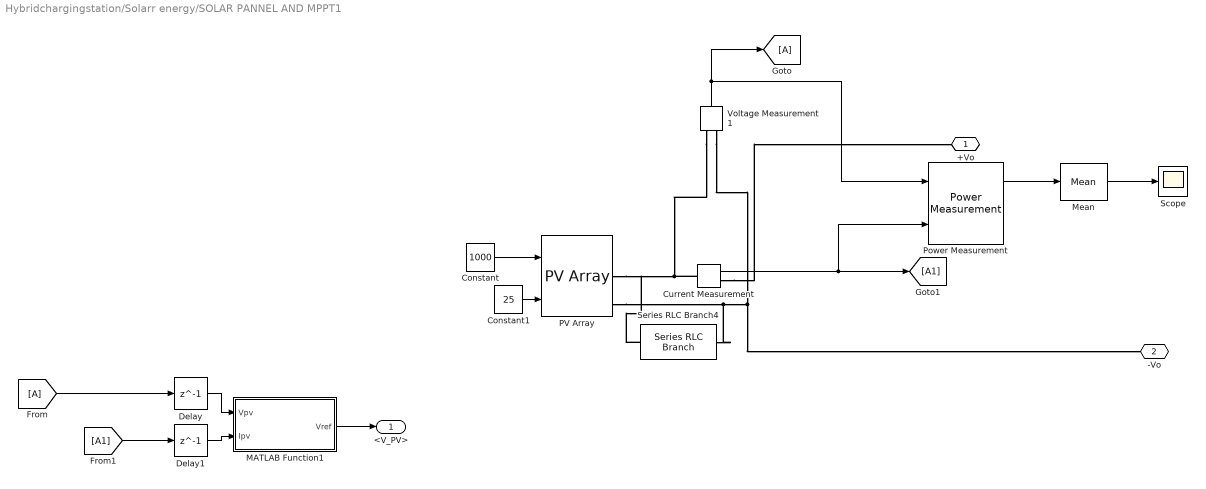
== system Hybridchargingstation/Solarr energy/SOLAR PANNEL AND MPPT1 ==
  Constant : Constant  Value=1000
  Constant1 : Constant  Value=25
  Current Measurement : spsCurrentMeasurementLib/Current Measurement  PhasorSimulation=off  OutputType=Complex  PSBequivalent=0
  Delay : Delay  DelayLength=1
  Delay1 : Delay  DelayLength=1
  From : From
  Goto : Goto
  MATLAB Function1 : MATLAB Function  TreatAsAtomicUnit=on
  Mean : spsMeanLib/Mean  Freq=50  Vinit=0  Ts=0
  PV Array : spsPVArrayLib/PV Array  Npar=10  Nser=15  PlotType=array @ 1000 W/m2 & specified temperatures  S_vec="[ 1000  500  100 ]"  Temp_C_vec="[  25  ]"  ModuleName=User-defined  PlotWhenSelected=off  Pm=220.5  Ncell=60  Voc=36.3  Isc=7.84  Vm=30  Im=7.35  beta_Voc_pc=-0.36099  alpha_Isc_pc=0.102  beta_Voc=-0.13104  alpha_Isc=0.0079968  IL=7.8464  I0=2.9192e-10  nI=0.98122  Rsh=295.3224  Rs=0.24205  RobustModel=off  RobustCellTemperature=313.3991  BAL=on  Tc=1e-6  Tfilter=5e-5
  Power Measurement : eePowerMeasurement/Power Measurement  LabelModeActiveChoice=Continuous  F=60  K=[0 1 2 3]  Ts=0
      settings: SourceProductBaseCode=PS
  Scope : Scope
  Series RLC Branch4 : spsSeriesRLCBranchLib/Series RLC Branch  LConnTagsString=__new0  RConnTagsString=__new0  BranchType=C  Resistance=1  Inductance=1e-3  SetiL0=off  InitialCurrent=0  Capacitance=1000e-6  Setx0=off  InitialVoltage=0  Measurements=None
  Voltage Measurement1 : spsVoltageMeasurementLib/Voltage Measurement  PhasorSimulation=off  OutputType=Complex  PSBequivalent=0
  +Vo : PMIOPort  Side=Right
  -Vo : PMIOPort  Port=2  Side=Right
  <V_PV> : Outport
  wires:
  Delay1/1 -> MATLAB Function1/2(Ipv)
  From/1 -> Delay/1
  Constant1/1 -> PV Array/2
  Constant/1 -> PV Array/1
  Delay/1 -> MATLAB Function1/1(Vpv)
  [A1] -> Delay1/1
  Voltage Measurement1/1 -> Power Measurement/1, Goto/1
  Current Measurement/1 -> Power Measurement/2, [A1]
  MATLAB Function1/1(Vref) -> <V_PV>/1
  Mean/1 -> Scope/1
  Power Measurement/1 -> Mean/1
  connections:
  Series RLC Branch4/LConn1 -- -Vo/RConn1 -- Voltage Measurement1/LConn2 -- PV Array/RConn2
  Current Measurement/RConn1 -- +Vo/RConn1
  Voltage Measurement1/LConn1 -- Current Measurement/LConn1 -- Series RLC Branch4/RConn1 -- PV Array/RConn1

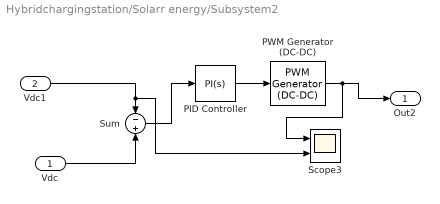
== system Hybridchargingstation/Solarr energy/Subsystem2 ==
  Vdc : Inport
  Vdc1 : Inport  Port=2
  PID Controller : slpidlib/PID Controller  Controller=PI  Form=Parallel  TimeDomain=Continuous-time  UseExternalTs=off  SampleTime=-1  IntegratorMethod=Forward Euler  FilterMethod=Forward Euler  ControllerParametersSource=internal  P=2  I=2  UseKiTs=off  D=0  N=100  UseFilter=on  TunerSelectOption=Transfer Function Based (PID Tuner App)  InitialConditionSource=internal  InitialConditionForIntegrator=0  InitialConditionForFilter=0  DifferentiatorICPrevScaledInput=0  ExternalReset=none  TrackingMode=off  Kt=1  LimitOutput=off  SatLimitsSource=internal  UpperSaturationLimit=inf  LowerSaturationLimit=-inf  LinearizeAsGain=on  AntiWindupMode=none  Kb=1  POutMin=[]  POutMax=[]  IOutMin=[]  IOutMax=[]  DOutMin=[]  DOutMax=[]  NOutMin=[]  NOutMax=[]  SumOutMin=[]  SumOutMax=[]  SaturationOutMin=[]  SaturationOutMax=[]  PParamMin=[]  PParamMax=[]  IParamMin=[]  IParamMax=[]  DParamMin=[]  DParamMax=[]  NParamMin=[]  NParamMax=[]  KbParamMin=[]  KbParamMax=[]  KtParamMin=[]  KtParamMax=[]  KbOutMin=[]  KbOutMax=[]  KtOutMin=[]  KtOutMax=[]  IntegratorOutMin=[]  IntegratorOutMax=[]  FilterOutMin=[]  FilterOutMax=[]  SumI1OutMin=[]  SumI1OutMax=[]  SumI2OutMin=[]  SumI2OutMax=[]  SumI3OutMin=[]  SumI3OutMax=[]  SumI4OutMin=[]  SumI4OutMax=[]  SumDOutMin=[]  SumDOutMax=[]  DifferentiatorOutMin=[]  DifferentiatorOutMax=[]  FilterDiffOutCoefMin=[]  FilterDiffOutCoefMax=[]  ReciprocalOutMin=[]  ReciprocalOutMax=[]  SumDenOutMin=[]  SumDenOutMax=[]  SumNumOutMin=[]  SumNumOutMax=[]  DivideOutMin=[]  DivideOutMax=[]  UdiffTsProdOutMin=[]  UdiffTsProdOutMax=[]  NTsProdOutMin=[]  NTsProdOutMax=[]  UintegralTsProdOutMin=[]  UintegralTsProdOutMax=[]  UngainTsProdOutMin=[]  UngainTsProdOutMax=[]  IntegratorContinuousStateAttributes=''  IntegratorStateMustResolveToSignalObject=off  IntegratorRTWStateStorageClass=Auto  FilterContinuousStateAttributes=''  FilterStateMustResolveToSignalObject=off  FilterRTWStateStorageClass=Auto  ParallelPVariant=InternalParameters  IdealPVariant=Disabled  IVariant=InternalParameters  DVariant=Disabled  IntegratorVariant=Continuous  SatVariant=Disabled  AWVariant=Passthrough  PCopyVariant=Disabled  TRVariant=Disabled  FdbkBlocksVariant=Forward  IdealPFdbkVariant=Disabled  SatFdbkVariant=Disabled  DerivativeFilterVariant=Disabled  NVariant=Disabled  NCopyVariant=Disabled_SignalSpec  FilterICVariant=Disabled  IntegratorICVariant=InternalICs  ExternalResetVariant=Disabled  TRSumVariant=Passthrough  SumFdbkVariant=Disabled  SumVariant=Sum_PI  TsampFilterVariant=InternalTs  TsampNgainVariant=Passthrough  TsampIntegralVariant=Passthrough  ExternalSaturationOutDataTypeStr=Inherit: Same as second input  aMode=0
  PWM Generator (DC-DC) : spsPWMGeneratorDCDCLib/PWM Generator (DC-DC)  Fsw=25000  Ts=0
  Scope3 : Scope  NumInputPorts=2
  Sum : Sum  Inputs=-+  InputSameDT=on  SaturateOnIntegerOverflow=on  OutDataTypeStr=Inherit: Same as first input
  Out2 : Outport
  wires:
  Sum/1 -> PID Controller/1
  Vdc/1 -> Sum/2
  PID Controller/1 -> PWM Generator (DC-DC)/1
  Vdc1/1 -> Scope3/2, Sum/1
  PWM Generator (DC-DC)/1 -> Scope3/1, Out2/1

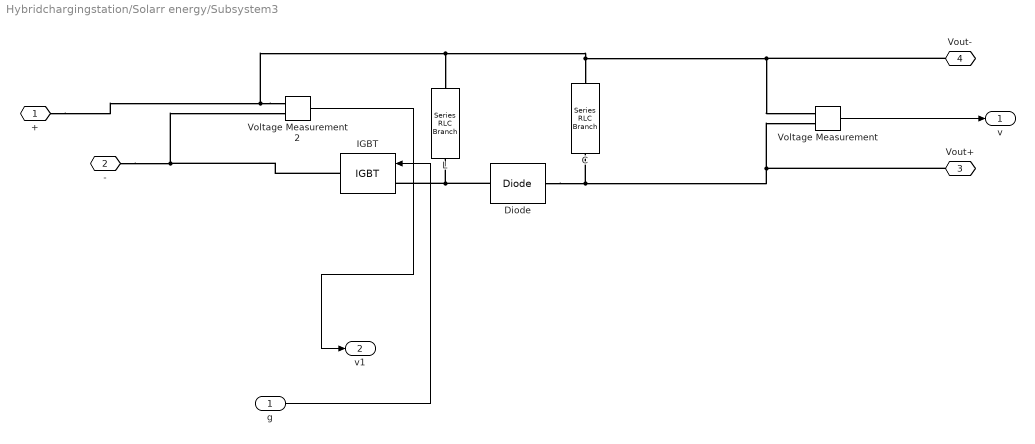
== system Hybridchargingstation/Solarr energy/Subsystem3 ==
  g : Inport
  C : spsSeriesRLCBranchLib/Series RLC Branch  LConnTagsString=__new0  RConnTagsString=__new0  BranchType=C  Resistance=1  Inductance=1e-3  SetiL0=off  InitialCurrent=0  Capacitance=4.7e-6  Setx0=off  InitialVoltage=0  Measurements=None
  Diode : spsDiodeLib/Diode  Ron=0.001  Lon=0  Vf=0.8  IC=0  UseSnubber=off  Rs=500  Cs=250e-9  Measurements=off
  IGBT : spsIGBTLib/IGBT  Ron=0.001  Lon=0  Vf=1  Tf=1e-6  Tt=2e-6  IC=0  Rs=1e5  Cs=inf  Measurements=off
  L : spsSeriesRLCBranchLib/Series RLC Branch  LConnTagsString=__new0  RConnTagsString=__new0  BranchType=L  Resistance=1  Inductance=2.4e-3  SetiL0=off  InitialCurrent=0  Capacitance=1e-6  Setx0=off  InitialVoltage=0  Measurements=None
  Voltage Measurement : spsVoltageMeasurementLib/Voltage Measurement  PhasorSimulation=off  OutputType=Complex  PSBequivalent=0
  Voltage Measurement2 : spsVoltageMeasurementLib/Voltage Measurement  PhasorSimulation=off  OutputType=Complex  PSBequivalent=0
  + : PMIOPort  Side=Left
  - : PMIOPort  Port=2  Side=Left
  Vout+ : PMIOPort  Port=3  Side=Right
  Vout- : PMIOPort  Port=4  Side=Right
  v : Outport
  v1 : Outport  Port=2
  wires:
  Voltage Measurement2/1 -> v1/1
  g/1 -> IGBT/1
  Voltage Measurement/1 -> v/1
  connections:
  Diode/RConn1 -- C/LConn1 -- Voltage Measurement/LConn1 -- Vout+/RConn1
  Voltage Measurement2/LConn1 -- +/RConn1 -- L/RConn1 -- Voltage Measurement/LConn2 -- Vout-/RConn1 -- C/RConn1
  Diode/LConn1 -- L/LConn1 -- IGBT/LConn1
  -/RConn1 -- Voltage Measurement2/LConn2 -- IGBT/RConn1

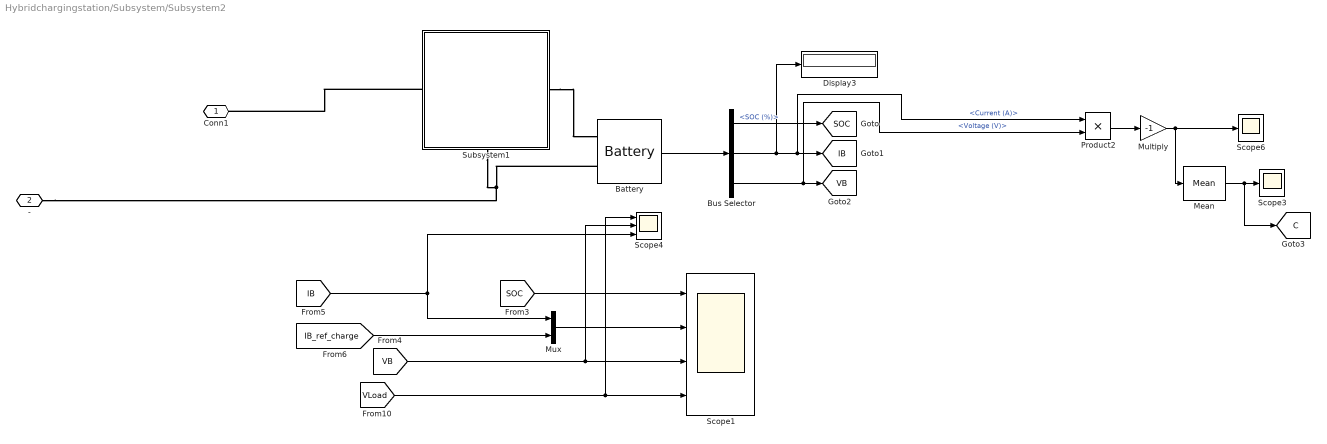
== system Hybridchargingstation/Subsystem/Subsystem2 ==
  Battery : spsBatteryLib/Battery  BatType=Lithium-Ion  ShowTempParam=off  ThermalPreset=no  ShowAgeParam=off  NomV=320  NomQ=93.93  SOC=45  Batt_Tr=1  PresetModel=on  MaxQ=93.93  MinV=240  FullV=372.4759  Dis_rate=40.8391  R=0.034068  Normal_OP=84.9454  expZone="[345.7235      4.614822]"  current=[6.5 13 32.5]  Units=Time  Tci=20  NomT=20  T2=-30  MaxQ2=4.8  FullV2=7.1  Normal_OP2=5.655  expZone2="[6.58           1]"  Rca=0.6  ti=2000  Dp=0  Neq0=0  Tsim=1e6  Ta1=25  Qeol=5.4*0.9  Reol=0.013333*1.2  Char_age=[2.3478, 3]  Dis_age=[2.3478, 10]  N1=1500  N2=10500  N3=1000  N4=1400  Ta2=45  N5=950
  Bus Selector : BusSelector  OutputSignals=SOC (%),Current (A),Voltage (V)
  Display3 : Display
  Mean : spsMeanLib/Mean  Freq=60  Vinit=0  Ts=0
  Multiply : Gain  Gain=-1
  Mux : Mux  Inputs=2
  Product2 : Product
  Scope1 : Scope  NumInputPorts=4
  Scope3 : Scope
  Scope4 : Scope  NumInputPorts=3
  Scope6 : Scope
  Subsystem1 : Subsystem
      settings: PortSchema="{\"entries\":[{\"content\":{\"sides\":[{\"content\":{\"connectorIds\":[\"LConn1\"]},\"type\":\"ConnectorPlacement.EquallySpacedRectSide\",\"uuid\":\"7a16d58d-936f-4863-9e65-620d6003398f\"},{\"content\":{\"connectorIds\":[\"RConn1\"],\"side\":\"RIGHT\"},\"type\":\"ConnectorPlacement.EquallySpacedRectSide\",\"uuid\":\"b355a268-5e94-4cff-ac50-21ca56722b08\"},{\"content\":{\"connectorIds\":[],\"side\":\"TOP\"},\"type\":\"ConnectorPlacement.EquallySpacedRectSide\",\"uuid\":\"4ff2972b-62ee-4777-9bce-190b6984e041\"},{\"content\":{\"connectorIds\":[\"RConn2\"],\"side\":\"BOTTOM\"},\"type\":\"ConnectorPlacement.EquallySpacedRectSide\",\"uuid\":\"3ea9ef25-7980-4110-b351-da5546fdc83f\"}]},\"type\":\"ConnectorPlacement.EquallySpacedConnector\",\"uuid\":\"9fe48545-d72f-43bd-bc54-8cb74ae97bd9\"}],\"packageUris\":[\"http://schema.mathworks.com/mf0/Connector/R2020b\"],\"version\":\"1.0\"}"
      mask Display: image('C:\Users\Sri Charan Reddy\Downloads\OIP (3).jpg'); % Use "Edit Image" on toolstrip to change.
  Conn1 : PMIOPort  Side=Left
  - : PMIOPort  Port=2  Side=Left
  tag scope: C=global, IB=global, SOC=global, VB=global
  wires:
  [SOC] -> Scope1/1
  Mux/1 -> Scope1/2
  Battery/1 -> Bus Selector/1
  [IB] -> Scope4/3, Mux/1
  Bus Selector/1 -> [SOC]  "<SOC (%)>"
  Bus Selector/2 -> Display3/1, Product2/1, [IB]  "<Current (A)>"
  [VLoad] -> Scope1/4, Scope4/1
  Multiply/1 -> Mean/1, Scope6/1
  [VB] -> Scope4/2, Scope1/3
  Bus Selector/3 -> Product2/2, [VB]  "<Voltage (V)>"
  [IB_ref_charge] -> Mux/2
  Product2/1 -> Multiply/1
  Mean/1 -> [C], Scope3/1
  connections:
  Subsystem1/LConn1 -- Conn1/RConn1
  Subsystem1/RConn2 -- -/RConn1 -- Battery/LConn2
  Subsystem1/RConn1 -- Battery/LConn1
